simulink model "canudas_goal2"  (R2012b)
settings: Solver=FixedStepDiscrete  StartTime=0.0  StopTime=Inf  FixedStep=0.033  RelTol=1e-3
values from neighbouring files (symbols this model uses):
  eps1 = 0.05    [param.m]
  eps2 = 2*pi*5/360    (= 0.0872664625997)    [param.m]
  K1 = 1.35    [param.m]
  K2 = 4.6    [param.m]
  thetar = pi    (= 3.14159265359)    [param.m]
  xr = 0    [param.m]
  yr = 0    [param.m]
libraries: simiam x5, simulink x3
settings Model: Creator=jdelacroix  LastModifiedBy=samati
settings DataIOCC: SignalLoggingSaveFormat=ModelDataLogs  SaveOutput=off  SaveTime=off
settings DebuggingCC: MultiTaskDSMMsg=warning  MultiTaskCondExecSysMsg=none  FcnCallInpInsideContextMsg=EnableAllAsWarning  StrictBusMsg=None
settings RTWCC: IncludeERTFirstTime=on
settings CodeAppCC: CustomSymbolStrType=$N$R$M_T  InternalIdentifier=Shortened
settings GRTTargetCC: CodeReplacementLibrary=None  CPPClassGenCompliant=on

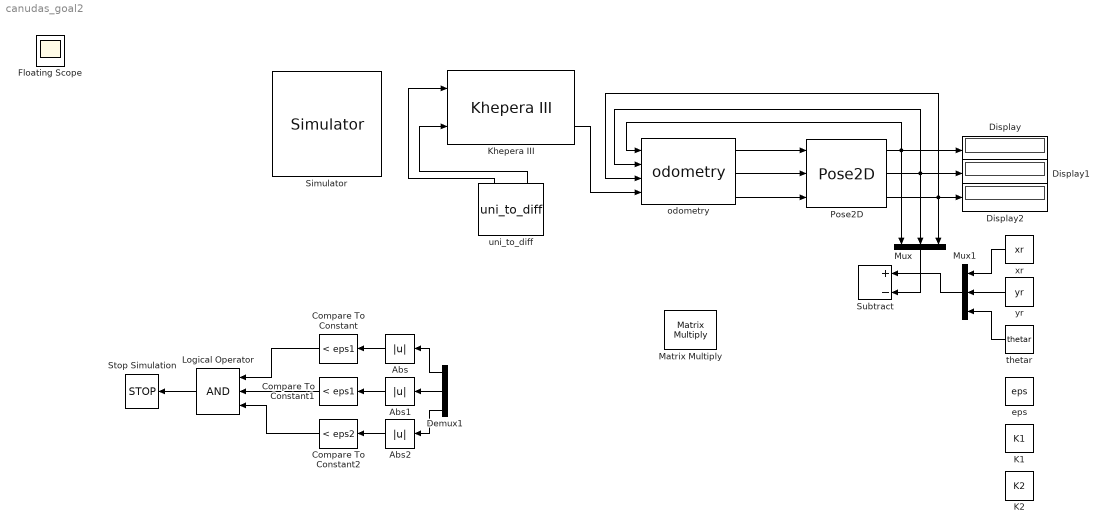
== system canudas_goal2 ==
  Abs : Abs
  Abs1 : Abs
  Abs2 : Abs
  Compare To Constant : simulink/Logic and Bit Operations/Compare To Constant  relop=<  const=eps1  OutDataTypeStr=boolean
  Compare To Constant1 : simulink/Logic and Bit Operations/Compare To Constant  relop=<  const=eps1  OutDataTypeStr=boolean
  Compare To Constant2 : simulink/Logic and Bit Operations/Compare To Constant  relop=<  const=eps2  OutDataTypeStr=boolean
  Demux1 : Demux  Outputs=3
  Display : Display
  Display1 : Display
  Display2 : Display
  K1 : Constant  Value=K1
  K2 : Constant  Value=K2
  Khepera III : simiam/Khepera III  x_0=0  y_0=0  theta_0=0  robot_id=1
  Logical Operator : Logic  Inputs=3  AllPortsSameDT=off  OutDataTypeStr=boolean
  Matrix Multiply : Product  Multiplication=Matrix(*)
  Mux : Mux  Inputs=3
  Mux1 : Mux  Inputs=3
  Pose2D : simiam/Pose2D  SystemSampleTime=-1
      link override Memory: X0=0
  Simulator : simiam/Simulator  Priority=1
  Stop Simulation : Stop
  Subtract : Sum  Inputs=+-
  eps : Constant  Value=eps
  odometry : simiam/odometry  wheel_radius=r  wheel_base_length=l  ticks_per_rev=2675
  thetar : Constant  Value=thetar
  uni_to_diff : simiam/uni_to_diff  wheel_radius=r  wheel_base_length=l
  xr : Constant  Value=xr
  yr : Constant  Value=yr
  Floating Scope : Scope
  wires:
  uni_to_diff/1 -> Khepera III/1
  uni_to_diff/2 -> Khepera III/2
  odometry/2 -> Pose2D/2
  odometry/1 -> Pose2D/1
  Khepera III/2 -> odometry/4
  Pose2D/1 -> Display/1, Mux/1, odometry/1
  Pose2D/2 -> Display1/1, odometry/2, Mux/2
  Pose2D/3 -> Display2/1, odometry/3, Mux/3
  odometry/3 -> Pose2D/3
  xr/1 -> Mux1/1
  yr/1 -> Mux1/2
  thetar/1 -> Mux1/3
  Logical Operator/1 -> Stop Simulation/1
  Compare To Constant1/1 -> Logical Operator/2
  Compare To Constant/1 -> Logical Operator/1
  Compare To Constant2/1 -> Logical Operator/3
  Demux1/1 -> Abs/1
  Abs/1 -> Compare To Constant/1
  Demux1/2 -> Abs1/1
  Abs1/1 -> Compare To Constant1/1
  Abs2/1 -> Compare To Constant2/1
  Demux1/3 -> Abs2/1
  Mux/1 -> Subtract/2
  Mux1/1 -> Subtract/1
